simulink model "Case1_UnifiedGFMandGFL_Indiviual_pu_2023a"  (R2023a)
settings: Solver=VariableStepAuto  StartTime=0  StopTime=10  RelTol=1e-3
model workspace (MAT data in the model file):
  Sbase = 1000000
  Vbase = 22000
libraries: simulink x5, spsGroundLib x4, spsControlledVoltageSourceLib x3, spsThreePhaseVIMeasurementLib x3, powerlib_extras x2, spsMeanLib x2, spsPLL3phLib x2, spsRMSLib x2, spsabctoAlphaBetaZeroLib x2, spsThreePhaseProgrammableVoltageSourceLib x1, spsThreePhaseSourceLib x1, spsThreePhaseSeriesRLCBranchLib x1
settings Model: SimulationMode=accelerator  Creator=wangxy  LastModifiedBy=wangxy
settings RTWCC: GPUComputeCapability=5.0

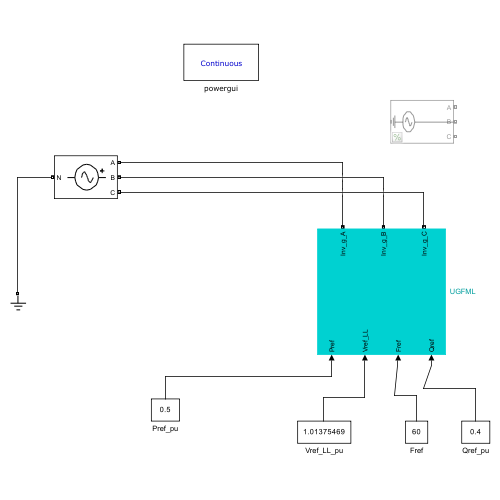
[thumbnail: Simulink's stored preview of the top-level diagram]
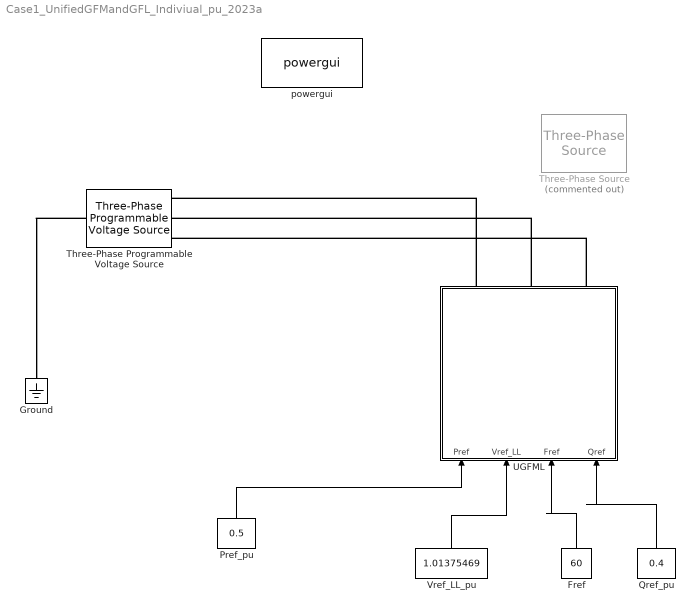
== system Case1_UnifiedGFMandGFL_Indiviual_pu_2023a ==
  Fref : Constant  Value=60
  Ground : spsGroundLib/Ground  LConnTagsString=a
  Pref_pu : Constant  Value=0.5
  Qref_pu : Constant  Value=0.4
  Three-Phase Programmable Voltage Source : spsThreePhaseProgrammableVoltageSourceLib/Three-Phase Programmable Voltage Source  PositiveSequence=[Vbase 0 60]  VariationEntity=Amplitude  VariationType=Step  VariationTypeAlt=Step  VariationStep=0.1  VariationRate=10  VariationMagnitude=0.3  VariationFrequency=2  VariationTiming=[4 8]  VariationPhaseA=off  Amplitudes=[1 0.8 1.2 1.0]  TimeValues=[0 0.1 0.15 0.2]  HarmonicGeneration=off  HarmonicA=[3 0.2 -25 0]  HarmonicB=[2 0.15 35 2]  Timing="[0.05  3]"  BusType=swing  Pref=0  Qref=0  Qmin=-inf  Qmax=inf
  Three-Phase Source : spsThreePhaseSourceLib/Three-Phase Source  Commented=on  InternalConnection=Yg  VoltagePhases=off  Voltage=Vbase  PhaseAngle=0  Voltage_phases=[25e3 25e3 25e3]/sqrt(3)  PhaseAngles_phases=[0 -120 +120]  Frequency=60  NonIdealSource=on  SpecifyImpedance=off  Resistance=0  Inductance=0  ShortCircuitLevel=100e6  BaseVoltage=Vbase  XRratio=7  BusType=swing  Pref=10e3  Qref=0  Prefabc=[10e3, 10e3, 10e3]  Qrefabc=[0, 0, 0]  Qmin=-inf  Qmax=inf
  UGFML : Subsystem
  Vref_LL_pu : Constant  Value=1.01375469
  powergui : spspowerguiLib/powergui  Priority=1  SimulationMode=Continuous  SampleTime=1e-4  frequency=60  Iterations=50  frequencyindice=60  Pbase=100e3  ErrMax=0.0001  UnitsV=kV  UnitsW=kW  buscounter=0  FunctionMessages=off  echomessages=off  EnableUseOfTLC=off  CurrentSourceSwitches=off  DisableSnubberDevices=off  DisableRonSwitches=off  DisableVfSwitches=off  DisplayEquations=off  AutomaticDiscreteSolvers=off  SolverType=Tustin/Backward Euler (TBE)  Interpol=off  ExternalGateDelay=off  methode=off  Ts=0  x0status=blocks  SPID=off  SwTol=0  HookPort=off  NonlinearTolerance=1e-4  nMaxIteration=100  ContinueOnMaxIteration=off  RestoreLinks=warning  ResistiveCurrentMeasurement=off  Frange=[0:2:500]  Ylog=off  Xlog=on  ShowGrid=off  save=off  variable=ZData  structure=0  ZoomFFT=on  StartTime=0.0  cycles=1  DisplayStyle=1  fundamental=60  FreqAxis=off  MaxFrequency=1000  frequencyindicesteady=1  RmsSteady=1  display=off
  wires:
  Qref_pu/1 -> UGFML/4(Qref)
  Vref_LL_pu/1 -> UGFML/2(Vref_LL)
  Pref_pu/1 -> UGFML/1(Pref)
  Fref/1 -> UGFML/3(Fref)
  connections:
  UGFML/RConn2 -- Three-Phase Programmable Voltage Source/RConn2
  UGFML/RConn1 -- Three-Phase Programmable Voltage Source/RConn1
  UGFML/RConn3 -- Three-Phase Programmable Voltage Source/RConn3
  Three-Phase Programmable Voltage Source/LConn1 -- Ground/LConn1

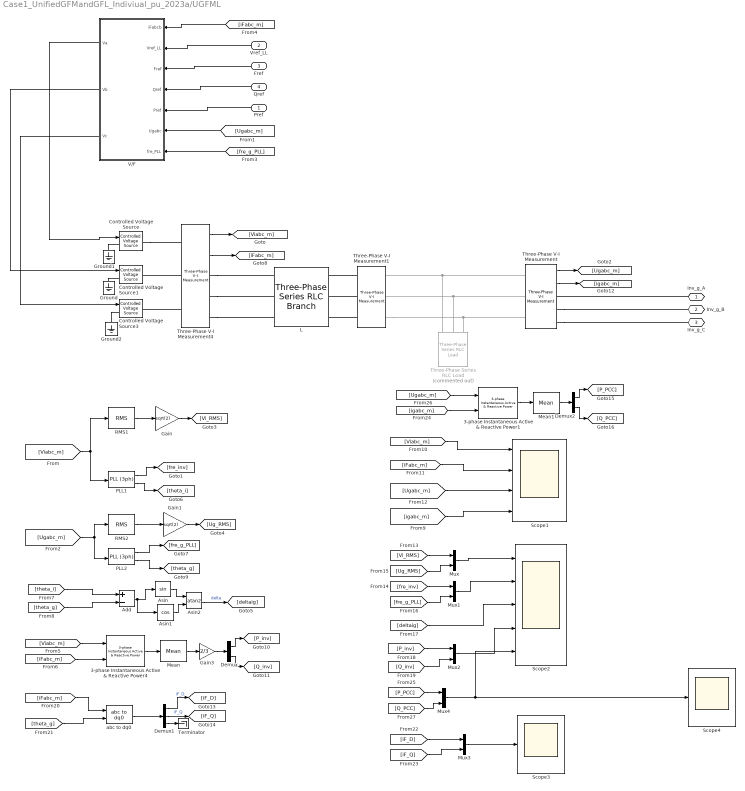
== system Case1_UnifiedGFMandGFL_Indiviual_pu_2023a/UGFML ==
  Pref : Inport
  Vref_LL : Inport  Port=2
  Fref : Inport  Port=3
  Qref : Inport  Port=4
  3-phase Instantaneous Active & Reactive Power1 : powerlib_extras/Measurements/3-phase  Instantaneous  Active & Reactive Power
  3-phase Instantaneous Active & Reactive Power4 : powerlib_extras/Measurements/3-phase  Instantaneous  Active & Reactive Power
  Add : Sum  Inputs=+-
  Asin : Trigonometry
  Asin1 : Trigonometry  Operator=cos
  Asin2 : Trigonometry  Operator=atan2
  Controlled Voltage Source : spsControlledVoltageSourceLib/Controlled Voltage Source  Initialize=on  Source_Type=DC  Amplitude=300  Phase=0  Frequency=60  Measurements=None
  Controlled Voltage Source1 : spsControlledVoltageSourceLib/Controlled Voltage Source  Initialize=on  Source_Type=DC  Amplitude=300  Phase=-120  Frequency=60  Measurements=None
  Controlled Voltage Source3 : spsControlledVoltageSourceLib/Controlled Voltage Source  Initialize=on  Source_Type=DC  Amplitude=300  Phase=120  Frequency=60  Measurements=None
  Demux : Demux  Outputs=2
  Demux1 : Demux  Outputs=3
  Demux2 : Demux  Outputs=2
  Gain : Gain  Gain=sqrt(2)
  Gain1 : Gain  Gain=sqrt(2)
  Gain3 : Gain  Gain=2/3
  Ground : spsGroundLib/Ground  LConnTagsString=a
  Ground1 : spsGroundLib/Ground  LConnTagsString=a
  Ground2 : spsGroundLib/Ground  LConnTagsString=a
  L : spsThreePhaseSeriesRLCBranchLib/Three-Phase Series RLC Branch  LConnTagsString=A|B|C  RConnTagsString=A|B|C  BranchType=RL  Resistance=0.01*Vbase^2/Sbase  Inductance=0.04*(Vbase^2/Sbase/377)  Capacitance=1.0  Measurements=None
  Mean : spsMeanLib/Mean  Freq=60  Vinit=0  Ts=5e-4
  Mean1 : spsMeanLib/Mean  Freq=60  Vinit=0  Ts=5e-4
  Mux{,1..4} (5 alike) : Mux  Inputs=2
  PLL1 : spsPLL3phLib/PLL (3ph)  Fmin=35  Par_Init=[0, 60]  ParK=[180, 3200, 1]  TcD=1e-4  MaxRateChangeFreq=12  FilterCutOffFreq=25  Ts=1e-5  AGC=on
  PLL2 : spsPLL3phLib/PLL (3ph)  Fmin=35  Par_Init=[0, 60]  ParK=[180, 3200, 1]  TcD=1e-4  MaxRateChangeFreq=12  FilterCutOffFreq=25  Ts=1e-5  AGC=on
  RMS1 : spsRMSLib/RMS  TrueRMS=on  Freq=60  RMSInit=1  Ts=5e-4
  RMS2 : spsRMSLib/RMS  TrueRMS=on  Freq=60  RMSInit=1  Ts=5e-4
  Scope1 : Scope  NumInputPorts=4
  Scope2 : Scope  NumInputPorts=5
  Scope3 : Scope
  Scope4 : Scope
  Terminator : Terminator
  Three-Phase Series RLC Load : spsThreePhaseSeriesRLCLoadLib/Three-Phase Series RLC Load  Commented=on  LConnTagsString=A|B|C  Configuration=Y (grounded)  NominalVoltage=22000  Vabc=[1e3 1e3 1e3]  Vabcp=[1e3 1e3 1e3]  NominalFrequency=60  UnbalancedPower=off  ActivePower=1e4  InductivePower=0  CapacitivePower=1e5  Pabc=[10e3 9e3 11e3]  QLabc=[100 90 110]  QCabc=[100 90 110]  Pabcp=[10e3 9e3 11e3]  QLabcp=[100 90 110]  QCabcp=[100 90 110]  Measurements=None  LoadType=constant Z
  Three-Phase V-I Measurement : spsThreePhaseVIMeasurementLib/Three-Phase V-I Measurement  VoltageMeasurement=phase-to-ground  SetLabelV=off  LabelV=Vabc  Vpu=on  VpuLL=off  CurrentMeasurement=yes  SetLabelI=off  LabelI=Iabc  Ipu=on  Pbase=Sbase  Vbase=Vbase  OutputType=Complex  PhasorSimulation=off  PSBequivalent=0
  Three-Phase V-I Measurement1 : spsThreePhaseVIMeasurementLib/Three-Phase V-I Measurement  VoltageMeasurement=no  SetLabelV=off  LabelV=Vabc  Vpu=off  VpuLL=off  CurrentMeasurement=no  SetLabelI=off  LabelI=Iabc  Ipu=off  Pbase=1e5  Vbase=380  OutputType=Complex  PhasorSimulation=off  PSBequivalent=0
  Three-Phase V-I Measurement4 : spsThreePhaseVIMeasurementLib/Three-Phase V-I Measurement  VoltageMeasurement=phase-to-ground  SetLabelV=off  LabelV=u  Vpu=on  VpuLL=off  CurrentMeasurement=yes  SetLabelI=off  LabelI=iFabcp3  Ipu=on  Pbase=Sbase  Vbase=Vbase  OutputType=Complex  PhasorSimulation=off  PSBequivalent=0
  V/F : Subsystem
  abc to dq0 : spsabctodq0Lib/abc to dq0  Alignment=90 degrees behind phase A axis
  Inv_g_A : PMIOPort  Side=Right
  Inv_g_B : PMIOPort  Port=2  Side=Right
  Inv_g_C : PMIOPort  Port=3  Side=Right
  wires:
  Three-Phase V-I Measurement/1 -> [Ugabc_m]
  3-phase Instantaneous Active & Reactive Power4/1 -> Mean/1
  Vref_LL/1 -> V/F/2(Vref_LL)
  V/F/2(Vb) -> Controlled Voltage Source1/1
  V/F/3(Vc) -> Controlled Voltage Source3/1
  Pref/1 -> V/F/5(Pref)
  Qref/1 -> V/F/4(Qref)
  Fref/1 -> V/F/3(Fref)
  RMS1/1 -> Gain/1
  Three-Phase V-I Measurement4/1 -> [Viabc_m]
  [Viabc_m] -> RMS1/1, PLL1/1
  PLL1/2 -> [theta_i]
  PLL1/1 -> [fre_inv]
  [Ugabc_m] -> V/F/6(Ugabc)
  [Ugabc_m] -> PLL2/1, RMS2/1
  RMS2/1 -> Gain1/1
  PLL2/2 -> [theta_g]
  PLL2/1 -> [fre_g_PLL]
  Three-Phase V-I Measurement4/2 -> [iFabc_m]
  [iFabc_m] -> V/F/1(iFabcb)
  [Viabc_m] -> 3-phase Instantaneous Active & Reactive Power4/1
  [iFabc_m] -> 3-phase Instantaneous Active & Reactive Power4/2
  Gain3/1 -> Demux/1
  Demux/1 -> [P_inv]
  Demux/2 -> [Q_inv]
  Three-Phase V-I Measurement/2 -> [igabc_m]
  [Viabc_m] -> Scope1/1
  [iFabc_m] -> Scope1/2
  [Ugabc_m] -> Scope1/3
  [igabc_m] -> Scope1/4
  [Vi_RMS] -> Mux/1
  [fre_inv] -> Mux1/1
  [Ug_RMS] -> Mux/2
  Mux/1 -> Scope2/1
  [fre_g_PLL] -> Mux1/2
  Mux1/1 -> Scope2/2
  [deltaig] -> Scope2/3
  [P_inv] -> Mux2/1
  [Q_inv] -> Mux2/2
  Mux2/1 -> Scope2/4
  Gain/1 -> [Vi_RMS]
  Gain1/1 -> [Ug_RMS]
  [fre_g_PLL] -> V/F/7(fre_PLL)
  [theta_i] -> Add/1
  Add/1 -> Asin/1, Asin1/1
  [theta_g] -> Add/2
  Asin/1 -> Asin2/1
  Asin1/1 -> Asin2/2
  Asin2/1 -> [deltaig]  "delta"
  [iFabc_m] -> abc to dq0/1
  [theta_g] -> abc to dq0/2
  abc to dq0/1 -> Demux1/1
  Demux1/3 -> Terminator/1
  Demux1/1 -> [iF_D]  "iF_D"
  Demux1/2 -> [iF_Q]  "iF_Q"
  [iF_D] -> Mux3/1
  [iF_Q] -> Mux3/2
  Mux3/1 -> Scope3/1
  V/F/1(Va) -> Controlled Voltage Source/1
  Demux2/2 -> [Q_PCC]
  [Ugabc_m] -> 3-phase Instantaneous Active & Reactive Power1/1
  [igabc_m] -> 3-phase Instantaneous Active & Reactive Power1/2
  Mean1/1 -> Demux2/1
  Demux2/1 -> [P_PCC]
  3-phase Instantaneous Active & Reactive Power1/1 -> Mean1/1
  [P_PCC] -> Mux4/1
  [Q_PCC] -> Mux4/2
  Mux4/1 -> Scope4/1, Scope2/5
  Mean/1 -> Gain3/1
  connections:
  Three-Phase V-I Measurement/RConn2 -- Inv_g_B/RConn1
  Three-Phase V-I Measurement4/LConn2 -- Controlled Voltage Source1/RConn1
  Controlled Voltage Source/RConn1 -- Three-Phase V-I Measurement4/LConn1
  Three-Phase V-I Measurement4/LConn3 -- Controlled Voltage Source3/RConn1
  Three-Phase Series RLC Load/LConn3 -- Three-Phase V-I Measurement1/RConn3 -- Three-Phase V-I Measurement/LConn3
  Three-Phase V-I Measurement/RConn3 -- Inv_g_C/RConn1
  Inv_g_A/RConn1 -- Three-Phase V-I Measurement/RConn1
  Three-Phase V-I Measurement4/RConn1 -- L/LConn1
  Three-Phase V-I Measurement4/RConn2 -- L/LConn2
  Three-Phase V-I Measurement4/RConn3 -- L/LConn3
  Controlled Voltage Source1/LConn1 -- Ground/LConn1
  Three-Phase Series RLC Load/LConn2 -- Three-Phase V-I Measurement1/RConn2 -- Three-Phase V-I Measurement/LConn2
  Three-Phase Series RLC Load/LConn1 -- Three-Phase V-I Measurement1/RConn1 -- Three-Phase V-I Measurement/LConn1
  Three-Phase V-I Measurement1/LConn1 -- L/RConn1
  Three-Phase V-I Measurement1/LConn2 -- L/RConn2
  Three-Phase V-I Measurement1/LConn3 -- L/RConn3
  Controlled Voltage Source/LConn1 -- Ground1/LConn1
  Controlled Voltage Source3/LConn1 -- Ground2/LConn1

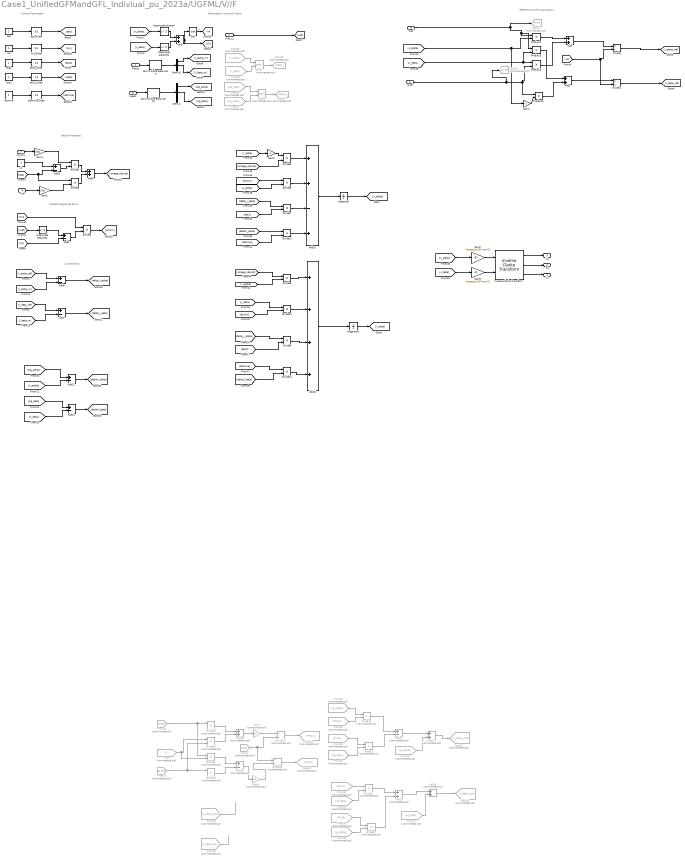
== system Case1_UnifiedGFMandGFL_Indiviual_pu_2023a/UGFML/V//F ==
  note: Natural Frequency
  note: Voltage Mangnitude Errror
  note: Current Error
  note: Control Parameters
  note: Parameters, Input and Output
  note: Reference Current Calculation
  iFabcb : Inport
  Vref_LL : Inport  Port=2
  Fref : Inport  Port=3
  Qref : Inport  Port=4
  Pref : Inport  Port=5
  Ugabc : Inport  Port=6
  fre_PLL : Inport  Port=7
  Add{,1..2,4} (4 alike) : Sum
  Add10 : Sum  Inputs=++-+
  Add11 : Sum  Inputs=++++
  Add{3,5..7,12..13} (6 alike) : Sum  Inputs=+-
  Add{15,18..20} (4 alike) : Sum  Commented=on
  Add16 : Sum  Commented=on  Inputs=+-
  Add17 : Sum  Commented=on  Inputs=+-
  Atan1 : Trigonometry  Commented=on  Operator=atan2
  Atan2 : Trigonometry  Commented=on  Operator=atan2
  Demux : Demux  Outputs=3
  Demux1 : Demux  Outputs=3
  Divide : Product  Inputs=*/
  Divide1 : Product  Inputs=*/
  Divide{2..12} (11 alike) : Product  Inputs=**
  Divide{13..16,19..22} (8 alike) : Product  Commented=on  Inputs=**
  Divide17 : Product  Commented=on  Inputs=*/
  Divide18 : Product  Commented=on  Inputs=/*
  From : From  Commented=on  GotoTag=X
  From1 : From  Commented=on  GotoTag=ug2
  From26 : From  Commented=on  GotoTag=Pref
  From27 : From  Commented=on  GotoTag=Qref
  From{28,32,36,51} (4 alike) : From  Commented=on  GotoTag=Ug_alpha
  From29 : From  Commented=on  GotoTag=PRQX
  From30 : From  Commented=on  GotoTag=PXQR
  From{31,34,37,52} (4 alike) : From  Commented=on  GotoTag=Ug_beta
  From33 : From  Commented=on  GotoTag=PRQX
  From35 : From  Commented=on  GotoTag=PXQR
  From38 : From  Commented=on  GotoTag=v_alpha_star
  From39 : From  Commented=on  GotoTag=v_beta_star
  From53 : From  Commented=on  GotoTag=v_alpha
  From54 : From  Commented=on  GotoTag=v_beta
  Gain1 : Gain  Gain=-1
  Gain3 : Gain  Gain=-1
  Gain4 : Gain  Gain=2*pi
  Gain5 : Gain  Gain=2*pi
  Gain6 : Gain  Gain=Vbase/sqrt(3)*sqrt(2)
  Gain7 : Gain  Commented=on  Gain=2/3
  Gain8 : Gain  Commented=on  Gain=2/3
  Gain9 : Gain  Gain=Vbase/sqrt(3)*sqrt(2)
  Gamma : Constant
  Gamma_Slider : simulink/Math Operations/Slider Gain  gain=0.0  low=0  high=10000
  Goto17 : Goto  Commented=on  GotoTag=Pref
  Goto18 : Goto  Commented=on  GotoTag=Qref
  Goto19 : Goto  Commented=on  GotoTag=PRQX
  Goto20 : Goto  Commented=on  GotoTag=PXQR
  Goto21 : Goto  Commented=on  GotoTag=v_alpha_star
  Goto22 : Goto  Commented=on  GotoTag=v_beta_star
  Goto27 : Goto  Commented=on  GotoTag=theta_g  TagVisibility=global
  Goto28 : Goto  Commented=on  GotoTag=theta_i  TagVisibility=global
  Integrator : Integrator  InitialCondition=0.8  LimitOutput=on  UpperSaturationLimit=10  LowerSaturationLimit=-10  ZeroCross=off
  Integrator1 : Integrator  InitialCondition=0.0001  LimitOutput=on  UpperSaturationLimit=10  LowerSaturationLimit=-10  ZeroCross=off
  Inverse Clarke Transform : mcbcontrolslib/Inverse Clarke Transform  PhaseInput=Two inputs  EnPowerInv=off
      settings: LibrarySourceBlock=mcblib/Controls/Math Transforms/Inverse Clarke Transform
  Magnitude Squared : Math  Operator=square
  Magnitude Squared1 : Math  Operator=square
  Magnitude Squared2 : Math  Operator=square
  Mu_Slider : simulink/Math Operations/Slider Gain  gain=0.0  low=0  high=30
  Product{1..4} (4 alike) : Product
  Sqrt : Sqrt
  abc to Alpha-Beta-Zero : spsabctoAlphaBetaZeroLib/abc to Alpha-Beta-Zero
  abc to Alpha-Beta-Zero1 : spsabctoAlphaBetaZeroLib/abc to Alpha-Beta-Zero
  eps : Constant
  eps_slider : simulink/Math Operations/Slider Gain  gain=0.0  low=0  high=1
  eta1 : Constant
  eta1_Slider : simulink/Math Operations/Slider Gain  gain=1.0  low=0  high=5
  eta2 : Constant
  eta2_Slider : simulink/Math Operations/Slider Gain  gain=1.0  low=0  high=5
  mu : Constant
  u1 : Constant
  Va : Outport
  Vb : Outport  Port=2
  Vc : Outport  Port=3
  tag scope: Vm=global
  wires:
  iFabcb/1 -> abc to Alpha-Beta-Zero/1
  Inverse Clarke Transform/1 -> Va/1
  Inverse Clarke Transform/2 -> Vb/1
  Inverse Clarke Transform/3 -> Vc/1
  abc to Alpha-Beta-Zero/1 -> Demux1/1
  Integrator1/1 -> [v_beta]
  Pref/1 -> Product3/1, Product1/1, Goto17/1
  [v_alpha] -> Gain1/1, Product1/2
  [v_beta] -> Product3/2, Product2/1
  Qref/1 -> Goto18/1, Product2/2, Product4/1
  Product1/1 -> Add/1
  Product2/1 -> Add/2
  Gain1/1 -> Product4/2
  Product3/1 -> Add1/1
  Product4/1 -> Add1/2
  [v_alpha] -> Magnitude Squared/1
  [v_beta] -> Magnitude Squared1/1
  Magnitude Squared/1 -> Add2/1
  Magnitude Squared1/1 -> Add2/2
  Add/1 -> Divide/1
  [v2] -> Divide/2, Divide1/2
  Add1/1 -> Divide1/1
  Divide/1 -> [i_alpha_ref]
  Divide1/1 -> [i_beta_ref]
  u1/1 -> Add3/1
  [eps] -> Divide3/1, Add3/2
  Add3/1 -> Divide2/2
  Fref/1 -> Gain5/1
  Divide2/1 -> Add4/1
  Divide3/1 -> Add4/2
  [v2] -> Add5/2
  Magnitude Squared2/1 -> Add5/1
  Add5/1 -> Divide4/2
  [errorV] -> Divide10/2
  [omega_natural] -> Divide5/2
  [v_beta] -> Gain3/1
  Gain3/1 -> Divide5/1
  [v_alpha] -> Divide6/2
  [i_alpha_ref] -> Add6/1
  [i_alpha_m] -> Add6/2
  [i_beta_ref] -> Add7/1
  Demux1/1 -> [i_alpha_m]
  Demux1/2 -> [i_beta_m]
  [i_beta_m] -> Add7/2
  Add6/1 -> [delta_i_alpha]
  Add7/1 -> [delta_i_beta]
  [delta_i_beta] -> Divide7/1
  [eta1] -> Divide7/2
  Divide7/1 -> Add10/3
  [delta_i_alpha] -> Divide8/1
  [eta2] -> Divide8/2
  Divide8/1 -> Add11/3
  Add10/1 -> Integrator/1
  Add11/1 -> Integrator1/1
  Gain5/1 -> Divide3/2
  Vref_LL/1 -> [vref]
  eta1_Slider/1 -> [eta1]
  eta1/1 -> eta1_Slider/1
  [vref] -> Magnitude Squared2/1
  [v_alpha] -> Divide9/2
  [v_beta] -> Divide10/1
  Divide5/1 -> Add10/1
  Divide9/1 -> Add10/2
  Divide6/1 -> Add11/1
  Divide10/1 -> Add11/2
  Ugabc/1 -> abc to Alpha-Beta-Zero1/1
  abc to Alpha-Beta-Zero1/1 -> Demux/1
  From38/1 -> ?
  [v_alpha] -> Add12/2
  From39/1 -> ?
  [v_beta] -> Add13/2
  Add12/1 -> [deltaV_alpha]
  Add13/1 -> [deltaV_beta]
  Divide11/1 -> Add10/4
  Divide12/1 -> Add11/4
  eta2/1 -> eta2_Slider/1
  eta2_Slider/1 -> [eta2]
  Gain4/1 -> Divide2/1
  Demux/1 -> [Ug_alpha]
  Demux/2 -> [Ug_beta]
  From26/1 -> Divide15/1, Divide13/1
  From/1 -> Divide15/2, Divide14/1
  From27/1 -> Divide16/1, Divide14/2
  Divide13/1 -> Add15/1
  Divide14/1 -> Add15/2
  Divide15/1 -> Add16/1
  Divide16/1 -> Add16/2
  Gain7/1 -> Divide17/1
  Gain8/1 -> Divide18/2
  From1/1 -> Divide18/1, Divide17/2
  Add15/1 -> Gain7/1
  Add16/1 -> Gain8/1
  Divide17/1 -> Goto19/1
  Divide18/1 -> Goto20/1
  From28/1 -> Divide19/1
  From29/1 -> Divide19/2
  From30/1 -> Divide20/1
  From31/1 -> Divide20/2
  Divide19/1 -> Add17/1
  Divide20/1 -> Add17/2
  Add17/1 -> Add18/1
  From32/1 -> Add18/2
  From33/1 -> Divide21/1
  From34/1 -> Divide21/2
  From35/1 -> Divide22/1
  From36/1 -> Divide22/2
  Divide21/1 -> Add19/1
  Divide22/1 -> Add19/2
  Add19/1 -> Add20/1
  From37/1 -> Add20/2
  Add18/1 -> Goto21/1
  Add20/1 -> Goto22/1
  [Ug_alpha] -> Add12/1
  [Ug_beta] -> Add13/1
  eps/1 -> eps_slider/1
  mu/1 -> Mu_Slider/1
  Mu_Slider/1 -> [mu]
  [mu] -> Divide4/1
  eps_slider/1 -> [eps]
  Gamma/1 -> Gamma_Slider/1
  Gamma_Slider/1 -> [Gamma]
  [Gamma] -> Divide11/2
  Divide4/1 -> [errorV]
  Add4/1 -> [omega_natural]
  [omega_natural] -> Divide6/1
  [errorV] -> Divide9/1
  Integrator/1 -> [v_alpha]
  [v_alpha] -> Gain6/1
  [Gamma] -> Divide12/1
  [deltaV_alpha] -> Divide11/1
  [deltaV_beta] -> Divide12/2
  [v_beta] -> Gain9/1
  Gain6/1 -> Inverse Clarke Transform/1
  Gain9/1 -> Inverse Clarke Transform/2
  From52/1 -> Atan2/1
  From51/1 -> Atan2/2
  Atan2/1 -> Goto27/1
  From53/1 -> Atan1/1
  From54/1 -> Atan1/2
  Atan1/1 -> Goto28/1
  fre_PLL/1 -> Gain4/1
  Sqrt/1 -> [Vm]  "Vm"
  Add2/1 -> [v2], Sqrt/1
